simulink model "OpenLoop"  (R2022a)
settings: Solver=VariableStepAuto  StartTime=0.0  StopTime=time  RelTol=1e-8
values from neighbouring files (symbols this model uses):
  beta = [0, (1/3)*-4/(-0.531), 1-((1/3)*-4/-0.531), 1]    [OpenLoopMain.m]
  Beta_x = [-0.2,-0.259,-0.275,-0.384, 0.261,-0.017, 0.248, 0.267, 0.259, 0.2]    [OpenLoopMain.m]
  Beta_y = [-0.5,-0.45,-0.406,-0.065,-1.031,0.095,-0.545,-0.374,-0.45,-0.5]    [OpenLoopMain.m]
  body_length = 0.7    [OpenLoopMain.m]
  g = 9.80665    [OpenLoopMain.m]
  I = 2.9    [OpenLoopMain.m]
  kD_flt = 224.2605    [OpenLoopMain.m]
  kD_knee = 0    [OpenLoopMain.m]
  kI_flt = -0.012    [OpenLoopMain.m]
  kI_knee = 303.1846    [OpenLoopMain.m]
  kP_flt = 1731.4    [OpenLoopMain.m]
  kP_knee = 1.1527e+03    (= 1152.7)    [OpenLoopMain.m]
  m = 33    [OpenLoopMain.m]
  N_flt = 4.3619    [OpenLoopMain.m]
  N_knee = 0    [OpenLoopMain.m]
  offset = 0.0295    [OpenLoopMain.m]
  r_2 = 0.3    [OpenLoopMain.m]
  T_air = (T_swing - T_stance)/2    (= 0.06)    [OpenLoopMain.m]
  T_swing = 0.22    [OpenLoopMain.m]
  th_i = -0.08    [OpenLoopMain.m]
  theta_1i = deg2rad(-101.5172)    [OpenLoopMain.m]
  theta_1i_B = theta_1i    [OpenLoopMain.m]
  theta_2i = deg2rad(80.4059)    [OpenLoopMain.m]
  y_i = 0.5 -(body_length/2)*sin(th_i)    [OpenLoopMain.m]
undefined symbols (not defined in the file or in its folder): X, Y, Z
libraries: sm_lib x34, nesl_utility x33, slpidlib x4
(part 2 of 2)

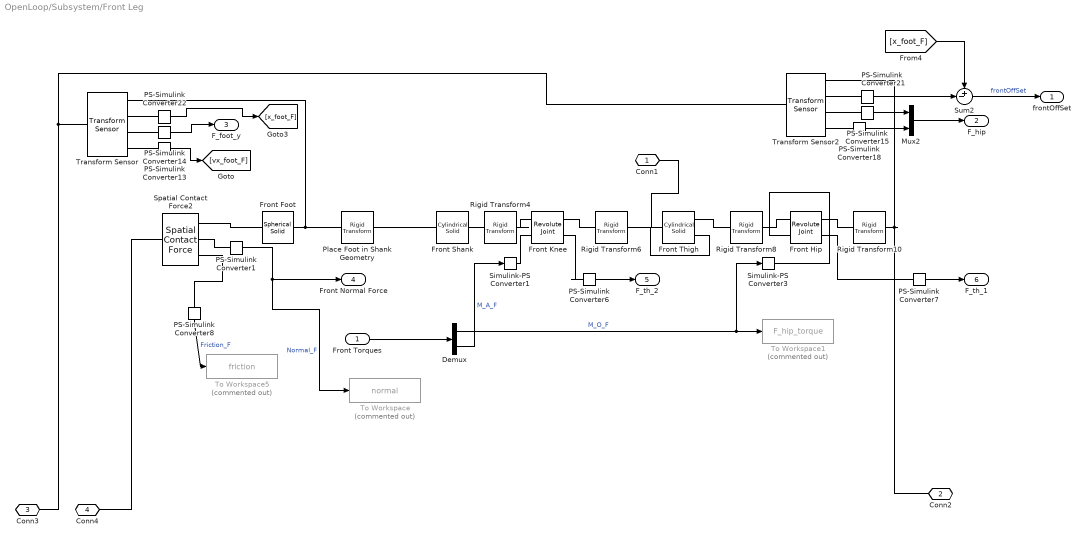
== system OpenLoop/Subsystem/Front Leg ==
  Front Torques : Inport
  Demux : Demux  Outputs=2
  Front Foot : sm_lib/Body Elements/Spherical Solid  GraphicAmbientColor=[0.15 0.15 0.15 1.0]  BasedOnType=Mass  CenterOfMass=[0 0 0]  CenterOfMassUnits=m  GraphicDiffuseColor=[0.0 0.0 0.0]  Density=1000  DensityUnits=kg/m^3  DoExposeReferenceFrame=on  GraphicEmissiveColor=[0.0 0.0 0.0 1.0]  ExportEntireGeometry=on  SerializedExposedGeometries=<ExposedGeometries><ExposedGeometry><RawGeometryId>entire</RawGeometryId><ExposedGeometryId>G</ExposedGeometryId></ExposedGeometry></ExposedGeometries>  SerializedFrames=<Frames/>  MarkerShape=Sphere  MarkerSize=10  GraphicType=FromGeometry  InertiaType=CalculateFromGeometry  Mass=1  MassUnits=g  MomentsOfInertia=[1 1 1]  MomentsOfInertiaUnits=kg*m^2  GraphicOpacity=1.0  ProductsOfInertia=[0 0 0]  ProductsOfInertiaUnits=kg*m^2  GraphicShininess=75  GraphicSpecularColor=[0.5 0.5 0.5 1.0]  SphereRadius=10  SphereRadiusUnits=mm  GraphicVisPropType=SimpleVisualProperties
  Front Hip : sm_lib/Joints/Revolute Joint  JointMode=Normal  SenseConstraintForce=off  SenseConstraintForceX=off  SenseConstraintForceY=off  SenseConstraintForceZ=off  SenseConstraintTorque=off  SenseConstraintTorqueX=off  SenseConstraintTorqueY=off  SenseConstraintTorqueZ=off  SenseTotalForce=off  SenseTotalForceX=off  SenseTotalForceY=off  SenseTotalForceZ=off  SenseTotalTorque=off  SenseTotalTorqueX=off  SenseTotalTorqueY=off  SenseTotalTorqueZ=off  CompositeWrenchDir=FollowerOnBase  CompositeWrenchFrame=BaseFrame  EquilibriumPosition=0  EquilibriumPositionUnits=deg  SpringStiffness=0  SpringStiffnessUnits=N*m/deg  DampingCoefficient=d_joint1  DampingCoefficientUnits=N*m/(deg/s)  TorqueActuationMode=InputTorque  MotionActuationMode=ComputedMotion  SensePosition=on  SenseVelocity=off  SenseAcceleration=off  SenseTorqueForce=off  SenseLowerLimitTorqueForce=off  SenseUpperLimitTorqueForce=off  LowerLimitSpecify=off  LowerLimitBound=-90  LowerLimitBoundUnits=deg  LowerLimitStiffness=1e4  LowerLimitStiffnessUnits=N*m/deg  LowerLimitDamping=10  LowerLimitDampingUnits=N*m/(deg/s)  LowerLimitTransitionRegionWidth=0.1  LowerLimitTransitionRegionWidthUnits=deg  UpperLimitSpecify=off  UpperLimitBound=90  UpperLimitBoundUnits=deg  UpperLimitStiffness=1e4  UpperLimitStiffnessUnits=N*m/deg  UpperLimitDamping=10  UpperLimitDampingUnits=N*m/(deg/s)  UpperLimitTransitionRegionWidth=0.1  UpperLimitTransitionRegionWidthUnits=deg  PositionTargetSpecify=on  PositionTargetPriority=High  PositionTargetValue=(theta_1i-th_i)  PositionTargetValueUnits=rad  VelocityTargetSpecify=off  VelocityTargetPriority=High  VelocityTargetValue=0  VelocityTargetValueUnits=deg/s
  Front Knee : sm_lib/Joints/Revolute Joint  JointMode=Normal  SenseConstraintForce=off  SenseConstraintForceX=off  SenseConstraintForceY=off  SenseConstraintForceZ=off  SenseConstraintTorque=off  SenseConstraintTorqueX=off  SenseConstraintTorqueY=off  SenseConstraintTorqueZ=off  SenseTotalForce=off  SenseTotalForceX=off  SenseTotalForceY=off  SenseTotalForceZ=off  SenseTotalTorque=off  SenseTotalTorqueX=off  SenseTotalTorqueY=off  SenseTotalTorqueZ=off  CompositeWrenchDir=FollowerOnBase  CompositeWrenchFrame=BaseFrame  EquilibriumPosition=0  EquilibriumPositionUnits=deg  SpringStiffness=0  SpringStiffnessUnits=N*m/deg  DampingCoefficient=d_joint2  DampingCoefficientUnits=N*m/(deg/s)  TorqueActuationMode=InputTorque  MotionActuationMode=ComputedMotion  SensePosition=on  SenseVelocity=off  SenseAcceleration=off  SenseTorqueForce=off  SenseLowerLimitTorqueForce=off  SenseUpperLimitTorqueForce=off  LowerLimitSpecify=off  LowerLimitBound=-90  LowerLimitBoundUnits=deg  LowerLimitStiffness=1e4  LowerLimitStiffnessUnits=N*m/deg  LowerLimitDamping=10  LowerLimitDampingUnits=N*m/(deg/s)  LowerLimitTransitionRegionWidth=0.1  LowerLimitTransitionRegionWidthUnits=deg  UpperLimitSpecify=off  UpperLimitBound=90  UpperLimitBoundUnits=deg  UpperLimitStiffness=1e4  UpperLimitStiffnessUnits=N*m/deg  UpperLimitDamping=10  UpperLimitDampingUnits=N*m/(deg/s)  UpperLimitTransitionRegionWidth=0.1  UpperLimitTransitionRegionWidthUnits=deg  PositionTargetSpecify=on  PositionTargetPriority=Low  PositionTargetValue=theta_2i  PositionTargetValueUnits=rad  VelocityTargetSpecify=off  VelocityTargetPriority=High  VelocityTargetValue=0  VelocityTargetValueUnits=deg/s
  Front Shank : sm_lib/Body Elements/Cylindrical Solid  GraphicAmbientColor=[0.15 0.15 0.15 1.0]  BasedOnType=Density  CenterOfMass=[0 0 0]  CenterOfMassUnits=m  GraphicDiffuseColor=[0.5 0.5 0.5]  CylinderLength=r_2  CylinderLengthUnits=m  CylinderRadius=0.01  CylinderRadiusUnits=m  Density=100  DensityUnits=kg/m^3  DoExposeReferenceFrame=on  GraphicEmissiveColor=[0.0 0.0 0.0 1.0]  ExportEntireGeometry=off  SerializedFrames=<Frames><Frame><Id>Frame1</Id><Value><Name>F1</Name><Origin><Source>GeometricFeature</Source><FeatureName>top surface</FeatureName></Origin><PrimaryAxis><DefinedDirection>+Z</DefinedDirection><Source>ReferenceFrame</Source><SourceDirection>+Z</SourceDirection><FeatureName></FeatureName></PrimaryAxis><SecondaryAxis><DefinedDirection>+X</DefinedDirection><Source>ReferenceFrame</Source><SourceDirection>+X</SourceDirection><FeatureName></FeatureName></SecondaryAxis></Value></Frame></Frames>  MarkerShape=Sphere  MarkerSize=10  GraphicType=FromGeometry  InertiaType=CalculateFromGeometry  Mass=1  MassUnits=g  MomentsOfInertia=[1 1 1]  MomentsOfInertiaUnits=kg*m^2  GraphicOpacity=1.0  ProductsOfInertia=[0 0 0]  ProductsOfInertiaUnits=kg*m^2  GraphicShininess=75  GraphicSpecularColor=[0.5 0.5 0.5 1.0]  GraphicVisPropType=SimpleVisualProperties
  Front Thigh : sm_lib/Body Elements/Cylindrical Solid  GraphicAmbientColor=[0.15 0.15 0.15 1.0]  BasedOnType=Density  CenterOfMass=[0 0 0]  CenterOfMassUnits=m  GraphicDiffuseColor=[0.5 0.5 0.5]  CylinderLength=r_1  CylinderLengthUnits=m  CylinderRadius=0.01  CylinderRadiusUnits=m  Density=100  DensityUnits=kg/m^3  DoExposeReferenceFrame=on  GraphicEmissiveColor=[0.0 0.0 0.0 1.0]  ExportEntireGeometry=off  SerializedFrames=<Frames><Frame><Id>Frame1</Id><Value><Name>F1</Name><Origin><Source>GeometricFeature</Source><FeatureName>top surface</FeatureName></Origin><PrimaryAxis><DefinedDirection>-X</DefinedDirection><Source>ReferenceFrame</Source><SourceDirection>+Z</SourceDirection><FeatureName></FeatureName></PrimaryAxis><SecondaryAxis><DefinedDirection>+Z</DefinedDirection><Source>ReferenceFrame</Source><SourceDirection>+X</SourceDirection><FeatureName></FeatureName></SecondaryAxis></Value></Frame><Frame><Id>Frame2</Id><Value><Name>F2</Name><Origin><Source>GeometricFeature</Source><FeatureName>bottom surface</FeatureName></Origin><PrimaryAxis><DefinedDirection>+Z</DefinedDirection><Source>ReferenceFrame</Source><SourceDirection>+Z</SourceDirection><FeatureName></FeatureName></PrimaryAxis><SecondaryAxis><DefinedDirection>+X</DefinedDirection><Source>ReferenceFrame</Source><SourceDirection>+X</SourceDirection><FeatureName></FeatureName></SecondaryAxis></Value></Frame></Frames>  MarkerShape=Sphere  MarkerSize=10  GraphicType=FromGeometry  InertiaType=CalculateFromGeometry  Mass=1  MassUnits=g  MomentsOfInertia=[1 1 1]  MomentsOfInertiaUnits=kg*m^2  GraphicOpacity=1.0  ProductsOfInertia=[0 0 0]  ProductsOfInertiaUnits=kg*m^2  GraphicShininess=75  GraphicSpecularColor=[0.5 0.5 0.5 1.0]  GraphicVisPropType=SimpleVisualProperties
  Mux2 : Mux  Inputs=2
  PS-Simulink Converter{1,6..8,13..15,18,21..22} (10 alike) : nesl_utility/PS-Simulink Converter  PhysicalDomain=network_engine_domain  SubClassName=ps_output  LeftPortType=input  RightPortType=output  PseudoPeriodic=off  Frequencies=[]  VectorFormat=1-D array  Unit=inherit  AffineConversion=off
      settings: SourceProductBaseCode=SS,PW,VE
  Place Foot in Shank Geometry : sm_lib/Frames and Transforms/Rigid Transform  TranslationMethod=Cartesian  TranslationStandardOffset=0  TranslationLengthUnit=m  TranslationStandardAxis=+Z  TranslationCartesianOffset=[0 0 r_2/2]  TranslationROffset=0  TranslationROffsetUnits=m  TranslationZOffset=0  TranslationZOffsetUnits=m  TranslationThetaOffset=0  TranslationThetaOffsetUnits=deg  RotationMethod=None  RotationAngleUnits=deg  RotationStandardAxis=+Z  RotationAngle=90  RotationArbitraryAxis=[0 0 1]  FollAlignAxisA=+X  BaseAlignAxisA=+Y  FollAlignAxisB=+Y  BaseAlignAxisB=+Z  RotationSequenceAxes=FollowerAxes  RotationSequence=XYX  RotationSequenceAngles=[0 0 0]  RotationSequenceAnglesUnits=deg  RotationMatrix=[1 0 0; 0 1 0; 0 0 1]
  Rigid Transform10 : sm_lib/Frames and Transforms/Rigid Transform  TranslationMethod=None  TranslationStandardOffset=0  TranslationLengthUnit=m  TranslationStandardAxis=+Z  TranslationCartesianOffset=[0 0 0]  TranslationROffset=0  TranslationROffsetUnits=m  TranslationZOffset=0  TranslationZOffsetUnits=m  TranslationThetaOffset=0  TranslationThetaOffsetUnits=deg  RotationMethod=StandardAxis  RotationAngleUnits=deg  RotationStandardAxis=+X  RotationAngle=90  RotationArbitraryAxis=[0 0 1]  FollAlignAxisA=+X  BaseAlignAxisA=+Y  FollAlignAxisB=+Y  BaseAlignAxisB=+Z  RotationSequenceAxes=FollowerAxes  RotationSequence=XYX  RotationSequenceAngles=[0 0 0]  RotationSequenceAnglesUnits=deg  RotationMatrix=[1 0 0; 0 1 0; 0 0 1]
  Rigid Transform4 : sm_lib/Frames and Transforms/Rigid Transform  TranslationMethod=None  TranslationStandardOffset=0  TranslationLengthUnit=m  TranslationStandardAxis=+Z  TranslationCartesianOffset=[0 0 0]  TranslationROffset=0  TranslationROffsetUnits=m  TranslationZOffset=0  TranslationZOffsetUnits=m  TranslationThetaOffset=0  TranslationThetaOffsetUnits=deg  RotationMethod=StandardAxis  RotationAngleUnits=deg  RotationStandardAxis=+X  RotationAngle=-90  RotationArbitraryAxis=[0 0 1]  FollAlignAxisA=+X  BaseAlignAxisA=+Y  FollAlignAxisB=+Y  BaseAlignAxisB=+Z  RotationSequenceAxes=FollowerAxes  RotationSequence=XYX  RotationSequenceAngles=[0 0 0]  RotationSequenceAnglesUnits=deg  RotationMatrix=[1 0 0; 0 1 0; 0 0 1]
  Rigid Transform6 : sm_lib/Frames and Transforms/Rigid Transform  TranslationMethod=None  TranslationStandardOffset=0  TranslationLengthUnit=m  TranslationStandardAxis=+Z  TranslationCartesianOffset=[0 0 0]  TranslationROffset=0  TranslationROffsetUnits=m  TranslationZOffset=0  TranslationZOffsetUnits=m  TranslationThetaOffset=0  TranslationThetaOffsetUnits=deg  RotationMethod=StandardAxis  RotationAngleUnits=deg  RotationStandardAxis=+X  RotationAngle=+90  RotationArbitraryAxis=[0 0 1]  FollAlignAxisA=+X  BaseAlignAxisA=+Y  FollAlignAxisB=+Y  BaseAlignAxisB=+Z  RotationSequenceAxes=FollowerAxes  RotationSequence=XYX  RotationSequenceAngles=[0 0 0]  RotationSequenceAnglesUnits=deg  RotationMatrix=[1 0 0; 0 1 0; 0 0 1]
  Rigid Transform8 : sm_lib/Frames and Transforms/Rigid Transform  TranslationMethod=None  TranslationStandardOffset=0  TranslationLengthUnit=m  TranslationStandardAxis=+Z  TranslationCartesianOffset=[0 0 0]  TranslationROffset=0  TranslationROffsetUnits=m  TranslationZOffset=0  TranslationZOffsetUnits=m  TranslationThetaOffset=0  TranslationThetaOffsetUnits=deg  RotationMethod=StandardAxis  RotationAngleUnits=deg  RotationStandardAxis=+X  RotationAngle=-90  RotationArbitraryAxis=[0 0 1]  FollAlignAxisA=+X  BaseAlignAxisA=+Y  FollAlignAxisB=+Y  BaseAlignAxisB=+Z  RotationSequenceAxes=FollowerAxes  RotationSequence=XYX  RotationSequenceAngles=[0 0 0]  RotationSequenceAnglesUnits=deg  RotationMatrix=[1 0 0; 0 1 0; 0 0 1]
  Simulink-PS Converter1 : nesl_utility/Simulink-PS Converter  PhysicalDomain=network_engine_domain  SubClassName=ps_input  LeftPortType=input  RightPortType=output  PseudoPeriodic=off  Frequencies=[]  NoiseDistribution=none  NoiseParameters=[]  Unit=1  AffineConversion=off  FilteringAndDerivatives=provide  SimscapeFilterOrder=1  InputFilterTimeConstant=0.001  UdotUserProvided=0
      settings: SourceProductBaseCode=SS,PW,VE
  Simulink-PS Converter3 : nesl_utility/Simulink-PS Converter  PhysicalDomain=network_engine_domain  SubClassName=ps_input  LeftPortType=input  RightPortType=output  PseudoPeriodic=off  Frequencies=[]  NoiseDistribution=none  NoiseParameters=[]  Unit=1  AffineConversion=off  FilteringAndDerivatives=provide  SimscapeFilterOrder=1  InputFilterTimeConstant=0.001  UdotUserProvided=0
      settings: SourceProductBaseCode=SS,PW,VE
  Spatial Contact Force2 : sm_lib/Forces and Torques/Spatial Contact Force  SenseContactBaseRotation=off  SenseContactBaseTranslation=off  CoefficientOfDynamicFriction=mu_k  CoefficientOfStaticFriction=mu_s  NormalDamping=contact_damping  NormalDampingUnits=N/(m/s)  SenseContactSignal=off  NormalStiffness=contact_stiffness  NormalStiffnessUnits=N/m  FrictionalCriticalVelocity=mu_vth  FrictionalCriticalVelocityUnits=m/s  ZeroCrossDetectContactStartAndEnd=off  SenseContactFollowerRotation=off  SenseContactFollowerTranslation=off  FrictionType=SmoothStickSlip  SenseFrictionalForceMagnitude=on  SenseNormalForceMagnitude=on  NormalForceType=SmoothSpringDamper  SenseNormalVelocity=off  SenseSeparationDistance=off  SenseTangentialVelocity=off  NormalTransitionRegionWidth=TransRegion  NormalTransitionRegionWidthUnits=m
  Sum2 : Sum  Inputs=+-|
  To Workspace : ToWorkspace  Commented=on  VariableName=normal  SampleTime=-1
  To Workspace1 : ToWorkspace  Commented=on  VariableName=F_hip_torque  SampleTime=-1
  To Workspace5 : ToWorkspace  Commented=on  VariableName=friction  SampleTime=-1
  Transform Sensor : sm_lib/Frames and Transforms/Transform Sensor  MeasurementFrame=World  SenseAngle=off  SenseAxis=off  SenseAngle1=off  SenseAngle2=off  SenseAngle3=off  SenseQ=off  SenseR=off  SenseOmegaX=off  SenseOmegaY=off  SenseOmegaZ=off  SenseOmega1=off  SenseOmega2=off  SenseOmega3=off  SenseQDot=off  SenseRDot=off  SenseAlphaX=off  SenseAlphaY=off  SenseAlphaZ=off  SenseAlpha1=off  SenseAlpha2=off  SenseAlpha3=off  SenseQDDot=off  SenseRDDot=off  SenseX=on  SenseY=off  SenseZ=on  SenseRad=off  SenseAzim=off  SenseDist=off  SenseInc=off  SenseXDot=on  SenseYDot=off  SenseZDot=off  SenseRadDot=off  SenseAzimDot=off  SenseDistDot=off  SenseIncDot=off  SenseXDDot=off  SenseYDDot=off  SenseZDDot=off  SenseRadDDot=off  SenseAzimDDot=off  SenseDistDDot=off  SenseIncDDot=off
  Transform Sensor2 : sm_lib/Frames and Transforms/Transform Sensor  MeasurementFrame=World  SenseAngle=off  SenseAxis=off  SenseAngle1=off  SenseAngle2=off  SenseAngle3=off  SenseQ=off  SenseR=off  SenseOmegaX=off  SenseOmegaY=off  SenseOmegaZ=off  SenseOmega1=off  SenseOmega2=off  SenseOmega3=off  SenseQDot=off  SenseRDot=off  SenseAlphaX=off  SenseAlphaY=off  SenseAlphaZ=off  SenseAlpha1=off  SenseAlpha2=off  SenseAlpha3=off  SenseQDDot=off  SenseRDDot=off  SenseX=on  SenseY=off  SenseZ=on  SenseRad=off  SenseAzim=off  SenseDist=off  SenseInc=off  SenseXDot=off  SenseYDot=off  SenseZDot=on  SenseRadDot=off  SenseAzimDot=off  SenseDistDot=off  SenseIncDot=off  SenseXDDot=off  SenseYDDot=off  SenseZDDot=off  SenseRadDDot=off  SenseAzimDDot=off  SenseDistDDot=off  SenseIncDDot=off
  Conn1 : PMIOPort  Side=Right
  Conn2 : PMIOPort  Port=2  Side=Right
  Conn3 : PMIOPort  Port=3  Side=Left
  Conn4 : PMIOPort  Port=4  Side=Left
  frontOffSet : Outport
  F_hip : Outport  Port=2
  F_foot_y : Outport  Port=3
  Front Normal Force : Outport  Port=4
  F_th_2 : Outport  Port=5
  F_th_1 : Outport  Port=6
  wires:
  PS-Simulink Converter14/1 -> F_foot_y/1
  PS-Simulink Converter1/1 -> Front Normal Force/1, To Workspace/1  "Normal_F"
  Mux2/1 -> F_hip/1
  Demux/1 -> To Workspace1/1, Simulink-PS Converter3/1  "M_O_F"
  [x_foot_F] -> Sum2/1
  Sum2/1 -> frontOffSet/1  "frontOffSet"
  PS-Simulink Converter21/1 -> Sum2/2
  PS-Simulink Converter8/1 -> To Workspace5/1  "Friction_F"
  PS-Simulink Converter7/1 -> F_th_1/1
  PS-Simulink Converter18/1 -> Mux2/2
  PS-Simulink Converter6/1 -> F_th_2/1
  PS-Simulink Converter13/1 -> [vx_foot_F]
  PS-Simulink Converter22/1 -> [x_foot_F]
  PS-Simulink Converter15/1 -> Mux2/1
  Front Torques/1 -> Demux/1
  Demux/2 -> Simulink-PS Converter1/1  "M_A_F"
  connections:
  PS-Simulink Converter13/LConn1 -- Transform Sensor/RConn4
  Transform Sensor2/RConn4 -- PS-Simulink Converter18/LConn1
  Transform Sensor2/LConn1 -- Conn3/RConn1 -- Transform Sensor/LConn1
  PS-Simulink Converter21/LConn1 -- Transform Sensor2/RConn2
  Rigid Transform10/LConn1 -- Front Hip/RConn1
  Front Foot/RConn1 -- Transform Sensor/RConn1 -- Place Foot in Shank Geometry/LConn1
  Front Knee/LConn2 -- Simulink-PS Converter1/RConn1
  PS-Simulink Converter22/LConn1 -- Transform Sensor/RConn2
  PS-Simulink Converter8/LConn1 -- Spatial Contact Force2/RConn3
  Spatial Contact Force2/RConn2 -- PS-Simulink Converter1/LConn1
  Front Shank/RConn1 -- Place Foot in Shank Geometry/RConn1
  Simulink-PS Converter3/RConn1 -- Front Hip/LConn2
  Rigid Transform10/RConn1 -- Conn2/RConn1 -- Transform Sensor2/RConn1
  Rigid Transform8/LConn1 -- Front Thigh/LConn1
  Transform Sensor2/RConn3 -- PS-Simulink Converter15/LConn1
  PS-Simulink Converter6/LConn1 -- Front Knee/RConn2
  PS-Simulink Converter14/LConn1 -- Transform Sensor/RConn3
  Front Thigh/RConn1 -- Conn1/RConn1
  PS-Simulink Converter7/LConn1 -- Front Hip/RConn2
  Front Thigh/LConn2 -- Rigid Transform6/RConn1
  Rigid Transform6/LConn1 -- Front Knee/RConn1
  Rigid Transform4/RConn1 -- Front Knee/LConn1
  Rigid Transform4/LConn1 -- Front Shank/LConn1
  Rigid Transform8/RConn1 -- Front Hip/LConn1
  Spatial Contact Force2/RConn1 -- Front Foot/LConn1
  Spatial Contact Force2/LConn1 -- Conn4/RConn1

== matlab function OpenLoop/MATLAB Function ==
  data: x input; theta input; F_th output; theta_dot input; th_1 input; th_2 input
function F_th = thetaForce(x,theta,theta_dot,th_1,th_2)
r_1 = 0.4;          % [m] thigh length
r_2 = 0.3;          % [m] shank length
kP_th = 25; %30 %25
kD_th = 15; %15 %11
th_des = -0.07;
th_dot_des = -0.5;
c_1 = cos(th_1+theta);
c_12 = cos(th_1+th_2+theta);

% x_foot = x_o + 0.2 + (0.7/2)*cos(theta); % instead of 0.2 try r_1*c_1 + r_2*c_12
x_foot = x(1) + r_1*c_1 + r_2*c_12 - (0.7/2)*cos(theta);

F_th = (1/(x(1)-x_foot))*kP_th*(theta - th_des) + kD_th*(theta_dot-th_dot_des);

== stateflow chart OpenLoop/Chart ==
  state FrontStance
    during:
    mod_time = time-touch_time_F;
    T_F = torque_profile_F(F_th_1,F_th_2,th,th_dot,x_y,x_y_dot,hip_height_F,mod_time,T_stance);
    tau_H = ((time-foot_lift_H+0.007)/T_swing);
    beta_H = [0, (1/3)*(foot_vel_H)/(-0.531), 1-((1/3)*-4/-0.531), 1];
    tau_H_mod = bezier(beta_H,tau_H);
    x_foot_des_H = bezier(Beta_x,tau_H_mod);
    y_foot_des_H = bezier(Beta_y,tau_H);
    [th_1_des_H, th_2_des_H] = inverse_kine(th, H_th_1, H_th_2, x_foot_des_H, y_foot_des_H);
    [T_H_1,T_H_2] = pos_control_H(th,H_th_1,H_th_2,th_1_des_H,th_2_des_H);
    T_H = [T_H_1;T_H_2];
    x_foot_des_F = bezier(Beta_x,0);
    y_foot_des_F = bezier(Beta_y,0);
    [th_1_des_F, th_2_des_F] = inverse_kine(th, F_th_1, F_th_2, x_foot_des_F, y_foot_des_F);
    [T_dumn1,T_dumn2] = pos_control_F(th, F_th_1, F_th_2, th_1_des_F, th_2_des_F);
  state Flight1
    during:
    tau_F = ((time - foot_lift_F+0.013)/T_swing);
    beta_F = [0, (1/3)*(foot_vel_F)/(-0.531), 1-((1/3)*-4/-0.531), 1];
    tau_F_mod = bezier(beta_F,tau_F);
    x_foot_des_F = bezier(Beta_x,tau_F_mod);
    y_foot_des_F = bezier(Beta_y,tau_F);
    [th_1_des_F, th_2_des_F] = inverse_kine(th, F_th_1, F_th_2, x_foot_des_F, y_foot_des_F);
    tau_H = (time-foot_lift_H)/T_swing;
    beta_H = [0, (1/3)*(foot_vel_H)/(-0.531), 1-((1/3)*-4/-0.531), 1];
    tau_H_mod = bezier(beta_H,tau_H);
    x_foot_des_H = bezier(Beta_x,tau_H_mod);
    y_foot_des_H = bezier(Beta_y,tau_H);
    [th_1_des_H, th_2_des_H] = inverse_kine(th, H_th_1, H_th_2, x_foot_des_H, y_foot_des_H);
    [T_F_1,T_F_2] = pos_control_F(th, F_th_1, F_th_2, th_1_des_F, th_2_des_F);
    T_F = [T_F_1;T_F_2];
    [T_H_1,T_H_2] = pos_control_H(th, H_th_1, H_th_2, th_1_des_H, th_2_des_H);
    T_H = [T_H_1;T_H_2];
  state [hip_torque,knee_torque] = pos_control_H(theta,th_1,th_2,th_1_d,th_2_d) [function]
  state [hip_torque,knee_torque] = pos_control_F(theta,th_1,th_2,th_1_d,th_2_d) [function]
  state BackStance
    during:
    mod_time = time-touch_time_H;
    tau_F = ((time - foot_lift_F+0.01)/T_swing);
    beta_F = [0, (1/3)*(foot_vel_F)/(-0.531), 1-((1/3)*-4/-0.531), 1];
    tau_F_mod = bezier(beta_F,tau_F);
    x_foot_des_F = bezier(Beta_x,tau_F_mod);
    y_foot_des_F = bezier(Beta_y,tau_F);
    [th_1_des_F, th_2_des_F] = inverse_kine(th, F_th_1, F_th_2, x_foot_des_F, y_foot_des_F);
    [T_F_1,T_F_2] = pos_control_F(th,F_th_1,F_th_2, th_1_des_F, th_2_des_F);
    T_F = [T_F_1;T_F_2];
    T_H = torque_profile_H(H_th_1,H_th_2,th,th_dot,x_y,x_y_dot,hip_height_H,mod_time,T_stance);
    x_foot_des_H = bezier(Beta_x,0);
    y_foot_des_H = bezier(Beta_y,0);
    [th_1_des_H, th_2_des_H] = inverse_kine(th, H_th_1, H_th_2, x_foot_des_H, y_foot_des_H);
    [T_dumn1,T_dumn2] = pos_control_H(th, H_th_1, H_th_2, th_1_des_H, th_2_des_H);
  state Pre_Impact
    during:
    tau_F = (T_air+T_stance+offset+time)/T_swing;
    tau_F_mod = bezier(beta,tau_F);
    x_foot_des_F = bezier(Beta_x,tau_F_mod);
    y_foot_des_F = bezier(Beta_y,tau_F);
    [th_1_des_F, th_2_des_F] = inverse_kine(th, F_th_1, F_th_2, x_foot_des_F, y_foot_des_F);
    [T_F_1,T_F_2] = pos_control_F(th, F_th_1, F_th_2, th_1_des_F, th_2_des_F);
    T_F = [T_F_1;T_F_2];
    tau_H = T_air/T_swing;
    tau_H_mod = bezier(beta, tau_H);
    x_foot_des_H = bezier(Beta_x,tau_H_mod);
    y_foot_des_H = bezier(Beta_y,tau_H);
    [th_1_des_H, th_2_des_H] = inverse_kine(th, H_th_1, H_th_2, x_foot_des_H, y_foot_des_H);
    [T_H_1,T_H_2] = pos_control_H(th, H_th_1, H_th_2, th_1_des_H, th_2_des_H);
    T_H = [T_H_1;T_H_2];
  state Flight2
    during:
    if (foot_vel_F > -2.75)
    foot_vel_F = -2.75;
    end
    tau_F = (time - foot_lift_F)/T_swing;
    beta_F = [0, (1/3)*(foot_vel_F)/(-0.531), 1-((1/3)*-4/-0.531), 1];
    tau_F_mod = bezier(beta_F,tau_F);
    x_foot_des_F = bezier(Beta_x,tau_F_mod);
    y_foot_des_F = bezier(Beta_y,tau_F);
    [th_1_des_F, th_2_des_F] = inverse_kine(th, F_th_1, F_th_2, x_foot_des_F, y_foot_des_F);
    [T_F_1,T_F_2] = pos_control_F(th,F_th_1,F_th_2, th_1_des_F, th_2_des_F);
    T_F = [T_F_1;T_F_2];
    tau_H = ((time-foot_lift_H+0.004)/T_swing);
    beta_H = [0, (1/3)*(foot_vel_H)/(-0.531), 1-((1/3)*-4/-0.531), 1];
    tau_H_mod = bezier(beta_H,tau_H);
    x_foot_des_H = bezier(Beta_x,tau_H_mod);
    y_foot_des_H = bezier(Beta_y,tau_H);
    [th_1_des_H, th_2_des_H] = inverse_kine(th, H_th_1, H_th_2, x_foot_des_H, y_foot_des_H);
    [T_H_1,T_H_2] = pos_control_H(th,H_th_1,H_th_2,th_1_des_H,th_2_des_H);
    T_H = [T_H_1;T_H_2];
  state FirstFlight
    during:
    if (foot_vel_F > -2.75)
    foot_vel_F = -2.75;
    end
    tau_F = (time - foot_lift_F)/T_swing;
    beta_F = [0, (1/3)*(foot_vel_F)/(-0.531), 1-((1/3)*-4/-0.531), 1];
    tau_F_mod = bezier(beta_F,tau_F);
    x_foot_des_F = bezier(Beta_x,tau_F_mod);
    y_foot_des_F = bezier(Beta_y,tau_F);
    [th_1_des_F, th_2_des_F] = inverse_kine(th, F_th_1, F_th_2, x_foot_des_F, y_foot_des_F);
    [T_F_1,T_F_2] = pos_control_F(th,F_th_1,F_th_2, th_1_des_F, th_2_des_F);
    T_F = [T_F_1;T_F_2];
    tau_H = ((time+T_air - touch_time_F+ 0.038)/T_swing);
    tau_H_mod = bezier(beta, tau_H);
    x_foot_des_H = bezier(Beta_x,tau_H_mod);
    y_foot_des_H = bezier(Beta_y,tau_H);
    [th_1_des_H, th_2_des_H] = inverse_kine(th, H_th_1, H_th_2, x_foot_des_H, y_foot_des_H);
    [T_H_1,T_H_2] = pos_control_H(th, H_th_1, H_th_2, th_1_des_H, th_2_des_H);
    T_H = [T_H_1;T_H_2];
  state FirstStance
    during:
    mod_time = time-touch_time_F;
    T_F = torque_profile_F(F_th_1,F_th_2,th,th_dot,x_y,x_y_dot,hip_height_F,mod_time,T_stance);
    tau_H = ((time+T_air - touch_time_F+0.03)/T_swing);
    tau_H_mod = bezier(beta, tau_H);
    x_foot_des_H = bezier(Beta_x,tau_H_mod);
    y_foot_des_H = bezier(Beta_y,tau_H);
    [th_1_des_H, th_2_des_H] = inverse_kine(th, H_th_1, H_th_2, x_foot_des_H, y_foot_des_H);
    [T_H_1,T_H_2] = pos_control_H(th,H_th_1,H_th_2,th_1_des_H,th_2_des_H);
    T_H = [T_H_1;T_H_2];
    x_foot_des_F = bezier(Beta_x,0);
    y_foot_des_F = bezier(Beta_y,0);
    [th_1_des_F, th_2_des_F] = inverse_kine(th, F_th_1, F_th_2, x_foot_des_F, y_foot_des_F);
    [T_dumn1,T_dumn2] = pos_control_F(th, F_th_1, F_th_2, th_1_des_F, th_2_des_F);
  Flight1 -> FrontStance : [fn_F>0]{touch_time_F = time;
      | mod_time = 0;
      | state = 1;}
  BackStance -> Flight1 : [(H_foot_y > 0.036) & (fn_H<1)]{foot_lift_H = time;
      | foot_vel_H = foot_x_dot_H;
      | state = 4;}
  FrontStance -> Flight2 : [(F_foot_y >0.036) & (fn_F <1)]{foot_lift_F = time;
      | foot_vel_F =  foot_x_dot_F;
      | state = 2;}
  (default) -> Pre_Impact : {state = 4;}
  Flight2 -> BackStance : [fn_H>0]{touch_time_H = time;
      | mod_time = 0;
      | n=n+1;
      | state = 3;}
  Pre_Impact -> FirstStance : [fn_F>0]{touch_time_F = time;
      | mod_time = 0;
      | state = 1;
      | amp_y_new = amp_y;}
  FirstFlight -> BackStance : [fn_H>0]{touch_time_H = time;
      | mod_time = 0;
      | n = 1;
      | state = 3;}
  FirstStance -> FirstFlight : [(F_foot_y >0.036) & (fn_F <1)]{foot_lift_F = time;
      | foot_vel_F = foot_x_dot_F;
      | state = 2;}
  data: th_1 function_input; th_2 function_input; theta function_input; theta_dot function_input; x function_input; x_dot function_input; hip_height function_input; t function_input; Torque function_output; T_sta function_input; P function_input; tau function_input; B function_output; theta function_input double size=1; th_1 function_input double size=1; th_2 function_input double size=1; th_1_d function_input double size=1; th_2_d function_input double size=1; hip_torque function_output; knee_torque function_output; theta function_input double size=1; th_1 function_input double size=1; th_2 function_input double size=1; th_1_d function_input double size=1; th_2_d function_input double size=1; hip_torque function_output; knee_torque function_output; theta function_input; theta_1g function_input; theta_2g function_input; foot_x_inv function_input; foot_y_inv function_input; theta_1 function_output; theta_2 function_output; th_1 function_input; th_2 function_input; theta function_input; theta_dot function_input; x function_input; x_dot function_input; hip_height function_input; t function_input; Torque function_output; T_sta function_input; F_th_1 input; F_th_2 input; th input; time input; T_stance constant double =T_stance; r_1 constant double =r_1; r_2 constant double =r_2; amp_x constant double =amp_x; amp_y constant double =amp_y; x_y input; x_y_dot input; x_dot_i constant double =x_dot_i; th_dot input; H_th_1 input; H_th_2 input; fn_F input; fn_H input; T_F output; T_H output; touch_time_F output size=1; touch_time_H output size=1; mod_time output size=1; F_foot_y input; H_foot_y input; hip_height_F input; hip_height_H input; T constant double =T; n local; theta_1i constant double =theta_1i; theta_2i constant double =theta_2i; T_F_1 local; T_F_2 local; theta_1i_B constant double =theta_1i_B; theta_2i_B constant double =theta_2i_B; T_H_1 local; T_H_2 local; Beta_x parameter; Beta_y parameter; T_swing parameter; x_foot_des_F local; y_foot_des_F local; foot_lift_F local; foot_lift_H local; tau_F local; tau_H local; T_air parameter; th_1_des_H output size=1; kP_flt parameter; kD_flt parameter; beta parameter; tau_H_mod local; beta_F local; beta_H local; tau_F_mod local; foot_x_dot_F input; foot_x_dot_H input; foot_vel_F local; foot_vel_H local; kI_flt parameter; N_flt parameter; th_1_des_F output size=1; T_dumn1 local; T_dumn2 local; state output size=1; x_foot_des_H output size=1; y_foot_des_H output size=1; th_2_des_H output size=1; dumb1 local; dumb2 local; th_2_des_F output size=1; offset parameter; body_length parameter; g parameter; m parameter; amp_y_new local
  function Torque = torque_profile_F(th_1,th_2,theta,theta_dot,x,x_dot,hip_height,t,T_sta):
    | function Torque = torque_profile_F(th_1,th_2,theta,theta_dot,x,x_dot,hip_height,t,T_sta)
    | 
    | s_1 = sin(th_1+theta);
    | c_1 = cos(th_1+theta);
    | s_12 = sin(th_1+th_2+theta);
    | c_12 = cos(th_1+th_2+theta);
    | 
    | J_T = [r_1*s_1 + r_2*s_12,  r_2*s_12
    |       -r_1*c_1 - r_2*c_12, -r_2*c_12]';
    |     
    | B_x = -amp_x*sin((pi()/T_sta)*t);
    | B_Y = amp_y_new*sin((pi()/T_sta)*t);
    | 
    | F = [B_x
    |      B_Y];
    | 
    | Torque = J_T*(F);
  function B = bezier(P,tau):
    | function B = bezier(P,tau)
    | %UNTITLED4 Summary of this function goes here
    | %   Detailed explanation goes here
    | n = length(P)-1;
    | B = zeros(length(tau));
    | for j = 1:length(tau)
    |     s_i = tau(j);
    |     if (s_i > 1)
    |         s_i = 1;
    |     end
    |     if (s_i<0)
    |         s_i = 0;
    |     end
    |     y = 0;
    |     for i = 0:n
    |         y = y + (nchoosek(n,i)*((1-s_i)^(n-i))*(s_i^(i))*P(i+1));
    |     end
    |     B(j) = y;
    | end
  function [theta_1 , theta_2] = inverse_kine(theta, theta_1g , theta_2g , foot_x_inv , foot_y_inv):
    | function [theta_1 , theta_2] = inverse_kine(theta, theta_1g , theta_2g , foot_x_inv , foot_y_inv)
    | 
    | % inverse_kine Inverse Kinematic Function
    | %   Takes two input guesses and returns the actual values values based off
    | %   of reducing error. Theta_2g and Theta_3g are the last calculated values
    | %   of theta 2 and theta 3 respectively that we will use as a point to
    | %   start iterating from. r_1 is the known magnitude vector 1 and theta_1
    | %   is the angle of that vector.
    | 
    | %% Inverse Kinematics for In Contact
    | 
    | % Initial Guesses
    | 
    | th_1 = theta_1g + theta; % Theta 1
    | th_2 = theta_2g; % Theta 2
    | 
    | % Our reasonable tolerance for position
    | epsilon = 5e-5;
    | 
    | % Setting a base epsilon to insure that code is read
    | epsilon1 = 1;
    | epsilon2 = 1;
    | 
    | % Setting a run-out timer
    | runs = 0;
    | 
    | %% Looping to converge on answer
    | 
    | while (epsilon1>= epsilon || epsilon2 >= epsilon && runs <= 10)
    |     
    |     runs = runs +1;
    |     
    |     % Defining Sin and Cos for our angles
    |     s12 = sin(th_2 + th_1);
    |     s1 = sin(th_1);
    |     c12 = cos(th_2 + th_1);
    |     c1 = cos(th_1);
    |     
    |     %Equations of Motion based off our angles
    |     delt_x = r_1*c1 + r_2*c12 - foot_x_inv;
    |     delt_y = r_1*s1 + r_2*s12 - foot_y_inv;
    |     
    |     %Partial derivatives
    |     dx_dth1 =-r_1*s1-r_2*s12;
    |     dx_dth2 =-s12*r_2;
    |     dy_dth1 =r_1*c1+r_2*c12;
    |     dy_dth2 =c12*r_2;
    |     
    |     %Defining Jacobian
    |     Jac = [dx_dth1 , dx_dth2 ; dy_dth1 , dy_dth2];
    |     
    |     %Setting old thetas and storing as "o"
    |     th_1o = th_1;
    |     th_2o = th_2;
    |     
    |     %Reguessing 
    |     xn_yn = [th_1;th_2] - ((Jac)\[delt_x;delt_y]);
    |     th_1 = xn_yn(1);
    |     th_2 = xn_yn(2);
    |     
    |     %Subtracting to refine our guesses
    |     epsilon1 = abs(th_1 - th_1o);
    |     epsilon2 = abs(th_2 - th_2o);
    |     
    | 
    | 
    | end
    | if (runs >= 10)
    |     
    |     error("inverse kinematics failed");
    | end
    | 
    | theta_1 = th_1;
    | theta_2 = th_2;
    | 
    | end
  function Torque = torque_profile_H(th_1,th_2,theta,theta_dot,x,x_dot,hip_height,t,T_sta):
    | function Torque = torque_profile_H(th_1,th_2,theta,theta_dot,x,x_dot,hip_height,t,T_sta)
    | 
    | s_1 = sin(th_1+theta);
    | c_1 = cos(th_1+theta);
    | s_12 = sin(th_1+th_2+theta);
    | c_12 = cos(th_1+th_2+theta);
    | 
    | J_T = [r_1*s_1 + r_2*s_12,  r_2*s_12
    |       -r_1*c_1 - r_2*c_12, -r_2*c_12]';
    |     
    | B_x = amp_x*sin((pi()/T_sta)*t);
    | B_Y = amp_y_new*sin((pi()/T_sta)*t);
    | 
    | F = [B_x
    |      B_Y];
    | 
    | Torque = J_T*(F);
